simulink model "MotorPosCntrl"  (R2020b)
settings: Solver=VariableStepAuto  StartTime=0.0  StopTime=0.2  RelTol=1e-3
undefined symbols (not defined in the file or in its folder): b, J, K, Kd, Ki, Kp, L, R
settings Model: Creator=BIDITA PAUL  LastModifiedBy=BIDITA PAUL

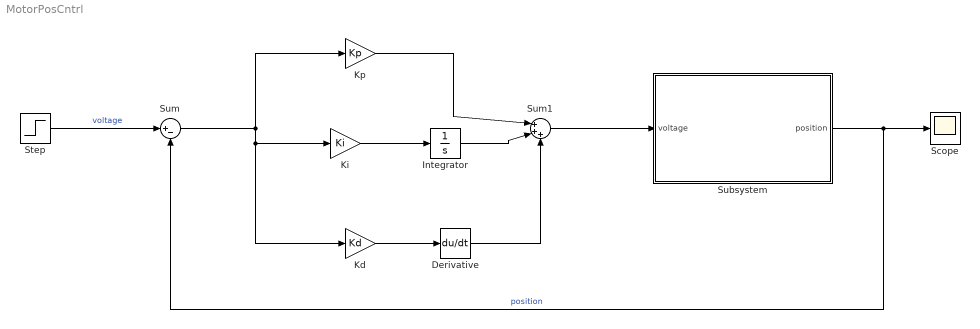
== system MotorPosCntrl ==
  Derivative : Derivative
  Integrator : Integrator
  Kd : Gain  Gain=Kd
  Ki : Gain  Gain=Ki
  Kp : Gain  Gain=Kp
  Scope : Scope
  Step : Step  Time=0  SampleTime=0
  Subsystem : Subsystem
  Sum : Sum  Inputs=|+-
  Sum1 : Sum  Inputs=|+++
  wires:
  Subsystem/1(position) -> Sum/2, Scope/1  "position"
  Step/1 -> Sum/1  "voltage"
  Sum/1 -> Ki/1, Kd/1, Kp/1
  Sum1/1 -> Subsystem/1(voltage)
  Integrator/1 -> Sum1/2
  Ki/1 -> Integrator/1
  Kp/1 -> Sum1/1
  Kd/1 -> Derivative/1
  Derivative/1 -> Sum1/3

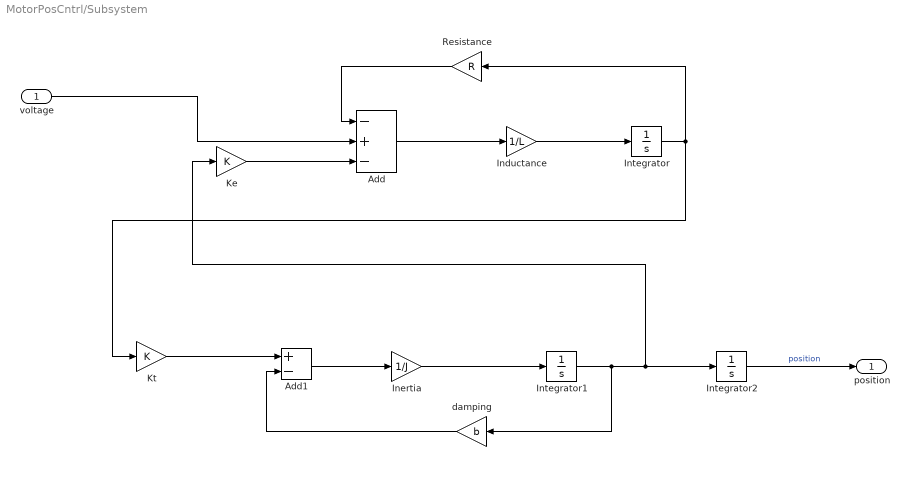
== system MotorPosCntrl/Subsystem ==
  voltage : Inport
  Add : Sum  Inputs=-+-
  Add1 : Sum  Inputs=+-
  Inductance : Gain  Gain=1/L
  Inertia : Gain  Gain=1/J
  Integrator : Integrator
  Integrator1 : Integrator
  Integrator2 : Integrator
  Ke : Gain  Gain=K
  Kt : Gain  Gain=K
  Resistance : Gain  Gain=R
  damping : Gain  Gain=b
  position : Outport
  wires:
  Integrator/1 -> Kt/1, Resistance/1
  Add/1 -> Inductance/1
  Resistance/1 -> Add/1
  Integrator1/1 -> damping/1, Ke/1, Integrator2/1
  Add1/1 -> Inertia/1
  Ke/1 -> Add/3
  damping/1 -> Add1/2
  Inductance/1 -> Integrator/1
  voltage/1 -> Add/2
  Inertia/1 -> Integrator1/1
  Kt/1 -> Add1/1
  Integrator2/1 -> position/1  "position"
